simulink model "Drone_old"  (R2021a)
settings: Solver=ode45  StartTime=0.0  StopTime=20  RelTol=1e-3
values from neighbouring files (symbols this model uses):
  B = 0.001    [Params.m]
  g = 9.81    [Params.m]
  I = [I_xx 0 0; 0 I_yy 0; 0 0 I_zz]    [Params.m]
  I_xx = 3*10^(-6)    (= 3e-06)    [Params.m]
  I_yy = 3*10^(-6)    (= 3e-06)    [Params.m]
  I_zz = 1*10^(-5)    (= 1e-05)    [Params.m]
  k = 0.01    [Params.m]
  kd = 0.01    [Params.m]
  kp_h = 218.061061208643    (= 218.061061209)    [Params.m]
  kp_r = 0.0160130109024398    (= 0.0160130109024)    [Params.m]    (also in pidsolver.m = kp)
  l = 0.225    [Params.m]
  m = 0.5    [Params.m]
  tau_d_h = 44.6853606001277    (= 44.6853606001)    [Params.m]
  tau_d_r = 0.00653126952336714    (= 0.00653126952337)    [Params.m]    (also in pidsolver.m = tau_i)
  tau_i_h = 110.138309959241    (= 110.138309959)    [Params.m]
  tau_i_r = 0.00736804577025044    (= 0.00736804577025)    [Params.m]    (also in pidsolver.m = tau_i)
  w_hover = 7.830229882    [Params.m]
libraries: pid_lib x1, vrlib x1
settings Model: Creator=Marcus  LastModifiedBy=Marcus

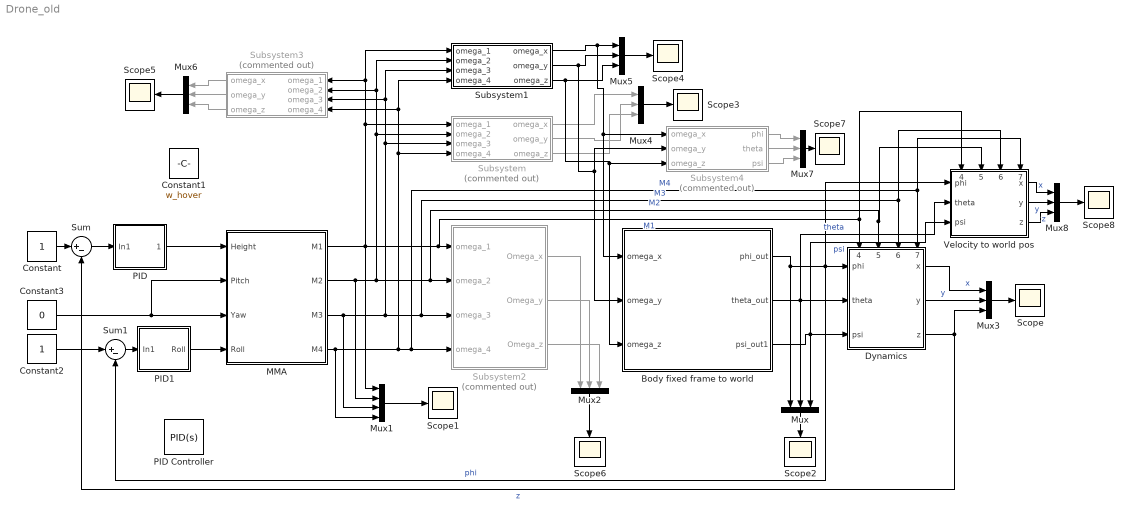
== system Drone_old ==
  Body fixed frame to world : Subsystem
  Constant : Constant  SampleTime=0.02
  Constant1 : Constant  Value=w_hover
  Constant2 : Constant  SampleTime=0.02
  Constant3 : Constant  Value=0  SampleTime=0.02
  Dynamics : Subsystem
      settings: PortSchema="{\"entries\":[{\"content\":{\"sides\":[{\"content\":{\"connectorIds\":[\"In1\",\"In2\",\"In3\"]},\"type\":\"ConnectorPlacement.EquallySpacedRectSide\",\"uuid\":\"56efaa7c-52a2-4b92-9bf3-e77850251265\"},{\"content\":{\"connectorIds\":[\"Out1\",\"Out2\",\"Out3\"],\"side\":\"RIGHT\"},\"type\":\"ConnectorPlacement.EquallySpacedRectSide\",\"uuid\":\"60524467-1949-4cc2-aa81-2e6d1e137057\"},{\"content\":{\"connectorIds\":[\"In4\",\"In5\",\"In6\",\"In7\"],\"side\":\"TOP\"},\"type\":\"ConnectorPlacement.EquallySpacedRectSide\",\"uuid\":\"33c04961-8bd6-41a2-b762-88d931b05d2b\"},{\"content\":{\"connectorIds\":[],\"side\":\"BOTTOM\"},\"type\":\"ConnectorPlacement.EquallySpacedRectSide\",\"uuid\":\"e0b8ebeb-9596-486e-9ed8-6640ac8c0b72\"}]},\"type\":\"ConnectorPlacement.EquallySpacedConnector\",\"uuid\":\"36d70e4f-9f0c-4c3e-93dc-a7f10cedf419\"}],\"packageUris\":[\"http://schema.mathworks.com/mf0/Connector/R2020b\"],\"version\":\"1.0\"}"
  MMA : Subsystem
  Mux{,2..8} (8 alike) : Mux  Inputs=3
  Mux1 : Mux
  PID : Subsystem
  PID Controller : pid_lib/PID Controller  Controller=PID  Form=Parallel  TimeDomain=Continuous-time  UseExternalTs=off  SampleTime=-1  IntegratorMethod=Forward Euler  FilterMethod=Forward Euler  ControllerParametersSource=internal  P=0.0160130109024398  I=0.00736804577025044  D=0.00653126952336714  UseFilter=on  N=1142.8279760416  TunerSelectOption=Transfer Function Based (PID Tuner App)  InitialConditionSource=internal  InitialConditionForIntegrator=0  InitialConditionForFilter=0  DifferentiatorICPrevScaledInput=0  ExternalReset=none  TrackingMode=off  Kt=1  LimitOutput=off  SatLimitsSource=internal  UpperSaturationLimit=inf  LowerSaturationLimit=-inf  LinearizeAsGain=on  AntiWindupMode=none  Kb=1  POutMin=[]  POutMax=[]  IOutMin=[]  IOutMax=[]  DOutMin=[]  DOutMax=[]  NOutMin=[]  NOutMax=[]  SumOutMin=[]  SumOutMax=[]  SaturationOutMin=[]  SaturationOutMax=[]  PParamMin=[]  PParamMax=[]  IParamMin=[]  IParamMax=[]  DParamMin=[]  DParamMax=[]  NParamMin=[]  NParamMax=[]  KbParamMin=[]  KbParamMax=[]  KtParamMin=[]  KtParamMax=[]  KbOutMin=[]  KbOutMax=[]  KtOutMin=[]  KtOutMax=[]  IntegratorOutMin=[]  IntegratorOutMax=[]  FilterOutMin=[]  FilterOutMax=[]  SumI1OutMin=[]  SumI1OutMax=[]  SumI2OutMin=[]  SumI2OutMax=[]  SumI3OutMin=[]  SumI3OutMax=[]  SumI4OutMin=[]  SumI4OutMax=[]  SumDOutMin=[]  SumDOutMax=[]  DifferentiatorOutMin=[]  DifferentiatorOutMax=[]  FilterDiffOutCoefMin=[]  FilterDiffOutCoefMax=[]  ReciprocalOutMin=[]  ReciprocalOutMax=[]  SumDenOutMin=[]  SumDenOutMax=[]  SumNumOutMin=[]  SumNumOutMax=[]  DivideOutMin=[]  DivideOutMax=[]  UdiffTsProdOutMin=[]  UdiffTsProdOutMax=[]  NTsProdOutMin=[]  NTsProdOutMax=[]  UintegralTsProdOutMin=[]  UintegralTsProdOutMax=[]  UngainTsProdOutMin=[]  UngainTsProdOutMax=[]  IntegratorContinuousStateAttributes=''  IntegratorStateMustResolveToSignalObject=off  IntegratorRTWStateStorageClass=Auto  FilterContinuousStateAttributes=''  FilterStateMustResolveToSignalObject=off  FilterRTWStateStorageClass=Auto  ParallelPVariant=InternalParameters  IdealPVariant=Disabled  IVariant=InternalParameters  DVariant=InternalParameters  IntegratorVariant=Continuous  SatVariant=Disabled  AWVariant=Passthrough  PCopyVariant=Disabled  TRVariant=Disabled  FdbkBlocksVariant=Forward  IdealPFdbkVariant=Disabled  SatFdbkVariant=Disabled  DerivativeFilterVariant=ContFilter  NVariant=InternalParameters  NCopyVariant=Disabled  FilterICVariant=InternalICsFilter  IntegratorICVariant=InternalICs  ExternalResetVariant=Disabled  TRSumVariant=Passthrough  SumFdbkVariant=Disabled  SumVariant=Sum_PID  TsampFilterVariant=InternalTs  TsampNgainVariant=Passthrough  TsampIntegralVariant=Passthrough  ExternalSaturationOutDataTypeStr=Inherit: Same as second input
  PID1 : Subsystem
  Scope{,1..8} (9 alike) : Scope
  Subsystem : Subsystem  Commented=on
  Subsystem1 : Subsystem
  Subsystem2 : Subsystem  Commented=on
  Subsystem3 : Subsystem  Commented=on
  Subsystem4 : Subsystem  Commented=on
  Sum : Sum  Inputs=|+-
  Sum1 : Sum  Inputs=|+-
  Velocity to world pos : Subsystem
      settings: PortSchema="{\"entries\":[{\"content\":{\"sides\":[{\"content\":{\"connectorIds\":[\"In1\",\"In2\",\"In3\"]},\"type\":\"ConnectorPlacement.EquallySpacedRectSide\",\"uuid\":\"56efaa7c-52a2-4b92-9bf3-e77850251265\"},{\"content\":{\"connectorIds\":[\"Out1\",\"Out2\",\"Out3\"],\"side\":\"RIGHT\"},\"type\":\"ConnectorPlacement.EquallySpacedRectSide\",\"uuid\":\"60524467-1949-4cc2-aa81-2e6d1e137057\"},{\"content\":{\"connectorIds\":[\"In4\",\"In5\",\"In6\",\"In7\"],\"side\":\"TOP\"},\"type\":\"ConnectorPlacement.EquallySpacedRectSide\",\"uuid\":\"33c04961-8bd6-41a2-b762-88d931b05d2b\"},{\"content\":{\"connectorIds\":[],\"side\":\"BOTTOM\"},\"type\":\"ConnectorPlacement.EquallySpacedRectSide\",\"uuid\":\"e0b8ebeb-9596-486e-9ed8-6640ac8c0b72\"}]},\"type\":\"ConnectorPlacement.EquallySpacedConnector\",\"uuid\":\"36d70e4f-9f0c-4c3e-93dc-a7f10cedf419\"}],\"packageUris\":[\"http://schema.mathworks.com/mf0/Connector/R2020b\"],\"version\":\"1.0\"}"
  wires:
  Body fixed frame to world/2(theta_out) -> Velocity to world pos/2(theta), Dynamics/2(theta), Mux/2  "theta"
  Subsystem2/3(Omega_z) -> Mux2/3
  Body fixed frame to world/1(phi_out) -> Mux/1, Velocity to world pos/1(phi), Sum1/2, Dynamics/1(phi)  "phi"
  Subsystem2/1(Omega_x) -> Mux2/1
  Body fixed frame to world/3(psi_out1) -> Velocity to world pos/3(psi), Dynamics/3(psi), Mux/3  "psi"
  Subsystem2/2(Omega_y) -> Mux2/2
  MMA/1(M1) -> Subsystem3/1(omega_1), Subsystem1/1(omega_1), Subsystem/1(omega_1), Dynamics/4(Input), Velocity to world pos/4(Input), Subsystem2/1(omega_1), Mux1/1  "M1"
  MMA/2(M2) -> Mux1/2, Subsystem3/2(omega_2), Subsystem1/2(omega_2), Subsystem/2(omega_2), Velocity to world pos/5(Input1), Dynamics/5(Input1), Subsystem2/2(omega_2)  "M2"
  MMA/3(M3) -> Mux1/3, Subsystem3/3(omega_3), Subsystem1/3(omega_3), Subsystem/3(omega_3), Subsystem2/3(omega_3), Dynamics/6(Input2), Velocity to world pos/6(Input2)  "M3"
  MMA/4(M4) -> Mux1/4, Subsystem3/4(omega_4), Subsystem1/4(omega_4), Subsystem/4(omega_4), Dynamics/7(Input3), Velocity to world pos/7(Input3), Subsystem2/4(omega_4)  "M4"
  Mux/1 -> Scope2/1
  Mux1/1 -> Scope1/1
  Constant/1 -> Sum/1
  Dynamics/2(y) -> Mux3/2  "y"
  Dynamics/1(x) -> Mux3/1  "x"
  Mux3/1 -> Scope/1
  Mux2/1 -> Scope6/1
  Subsystem/1(omega_x) -> Mux4/1
  Subsystem/2(omega_y) -> Mux4/2
  Subsystem/3(omega_z) -> Mux4/3
  Mux4/1 -> Scope3/1
  Mux5/1 -> Scope4/1
  Subsystem1/1(omega_x) -> Body fixed frame to world/1(omega_x), Subsystem4/1(omega_x), Mux5/1
  Subsystem1/2(omega_y) -> Body fixed frame to world/2(omega_y), Subsystem4/2(omega_y), Mux5/2
  Subsystem1/3(omega_z) -> Body fixed frame to world/3(omega_z), Subsystem4/3(omega_z), Mux5/3
  Mux6/1 -> Scope5/1
  Subsystem3/1(omega_x) -> Mux6/1
  Subsystem3/2(omega_y) -> Mux6/2
  Subsystem3/3(omega_z) -> Mux6/3
  Subsystem4/1(phi) -> Mux7/1
  Subsystem4/2(theta) -> Mux7/2
  Subsystem4/3(psi) -> Mux7/3
  Mux7/1 -> Scope7/1
  Dynamics/3(z) -> Sum/2, Mux3/3  "z"
  Constant2/1 -> Sum1/1
  Sum1/1 -> PID1/1(In1)
  PID1/1(Roll) -> MMA/4(Roll)
  Sum/1 -> PID/1(In1)
  PID/1(Height) -> MMA/1(Height)
  Mux8/1 -> Scope8/1
  Velocity to world pos/1(x) -> Mux8/1  "x"
  Velocity to world pos/2(y) -> Mux8/2  "y"
  Velocity to world pos/3(z) -> Mux8/3  "z"
  Constant3/1 -> MMA/2(Pitch), MMA/3(Yaw)

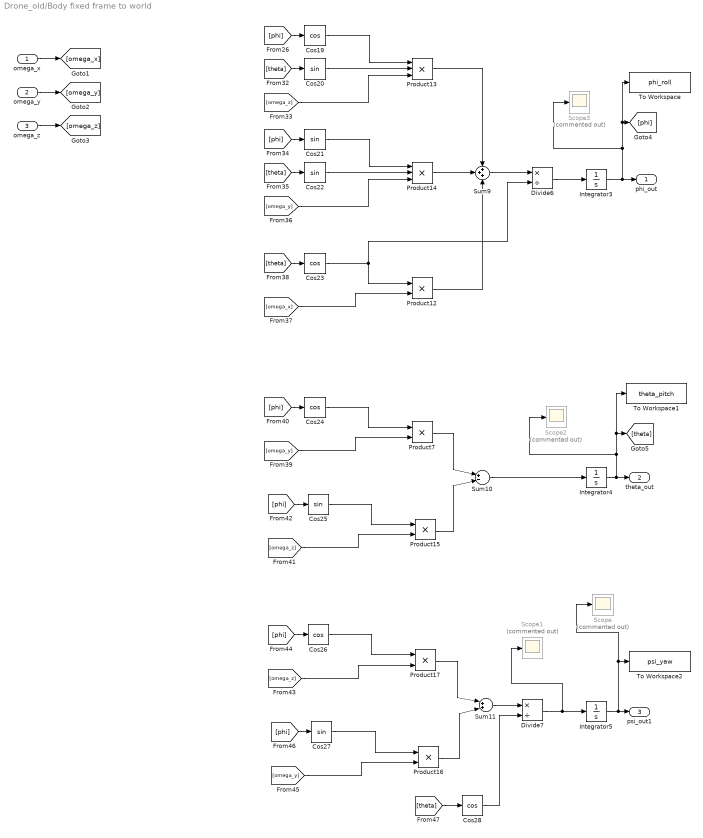
== system Drone_old/Body fixed frame to world ==
  omega_x : Inport
  omega_y : Inport  Port=2
  omega_z : Inport  Port=3
  Cos{19,23..24,26,28} (5 alike) : Trigonometry  Operator=cos
  Cos{20..22,25,27} (5 alike) : Trigonometry
  Divide6 : Product  Inputs=*/
  Divide7 : Product  Inputs=*/
  Integrator3 : Integrator
  Integrator4 : Integrator
  Integrator5 : Integrator
  Product{7,12,15..17} (5 alike) : Product
  Product13 : Product  Inputs=3
  Product14 : Product  Inputs=3
  Scope{,1..3} (4 alike) : Scope  Commented=on
  Sum10 : Sum  Inputs=|+-|
  Sum11 : Sum  Inputs=|++|
  Sum9 : Sum  Inputs=+++
  To Workspace : ToWorkspace  VariableName=phi_roll  SaveFormat=Timeseries  SampleTime=-1
  To Workspace1 : ToWorkspace  VariableName=theta_pitch  SaveFormat=Timeseries  SampleTime=-1
  To Workspace2 : ToWorkspace  VariableName=psi_yaw  SaveFormat=Timeseries  SampleTime=-1
  phi_out : Outport
  theta_out : Outport  Port=2
  psi_out1 : Outport  Port=3
  wires:
  omega_x/1 -> [omega_x]
  omega_y/1 -> [omega_y]
  omega_z/1 -> [omega_z]
  Cos19/1 -> Product13/1
  [phi] -> Cos19/1
  Cos20/1 -> Product13/2
  [theta] -> Cos20/1
  [omega_z] -> Product13/3
  Cos22/1 -> Product14/2
  [theta] -> Cos22/1
  [phi] -> Cos21/1
  Cos21/1 -> Product14/1
  [omega_y] -> Product14/3
  [omega_x] -> Product12/2
  [theta] -> Cos23/1
  Cos23/1 -> Product12/1, Divide6/2
  Product14/1 -> Sum9/2
  Product13/1 -> Sum9/1
  Product12/1 -> Sum9/3
  Sum9/1 -> Divide6/1
  Divide6/1 -> Integrator3/1
  Integrator3/1 -> Scope3/1, To Workspace/1, [phi], phi_out/1
  [omega_y] -> Product7/2
  Cos24/1 -> Product7/1
  [phi] -> Cos24/1
  [phi] -> Cos25/1
  Cos25/1 -> Product15/1
  [omega_z] -> Product15/2
  Product15/1 -> Sum10/2
  Product7/1 -> Sum10/1
  Sum10/1 -> Integrator4/1
  Integrator4/1 -> Scope2/1, To Workspace1/1, [theta], theta_out/1
  Product17/1 -> Sum11/1
  [phi] -> Cos26/1
  [omega_z] -> Product17/2
  Cos27/1 -> Product16/1
  [phi] -> Cos27/1
  Integrator5/1 -> Scope/1, To Workspace2/1, psi_out1/1
  [omega_y] -> Product16/2
  Cos26/1 -> Product17/1
  Product16/1 -> Sum11/2
  Sum11/1 -> Divide7/1
  Cos28/1 -> Divide7/2
  [theta] -> Cos28/1
  Divide7/1 -> Scope1/1, Integrator5/1

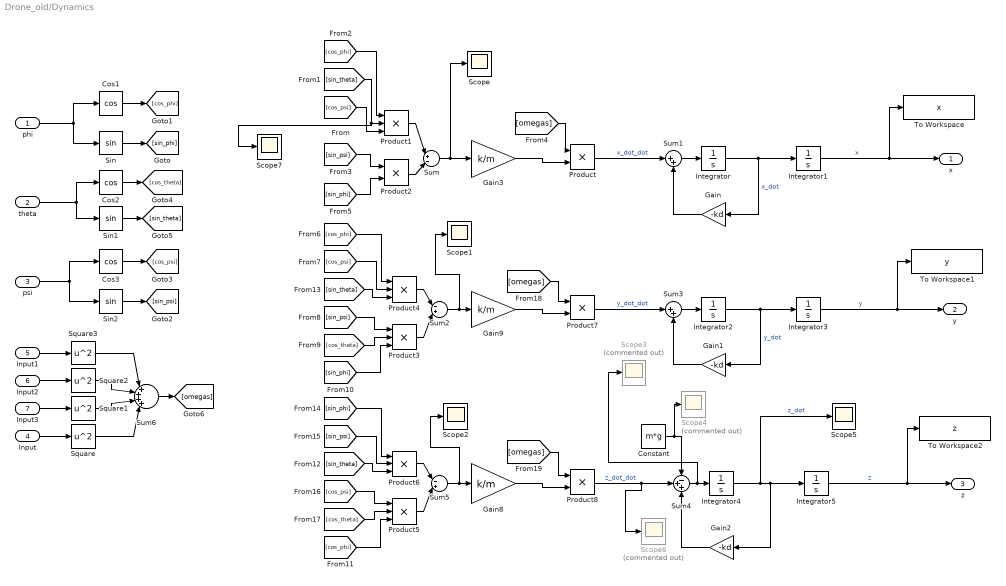
== system Drone_old/Dynamics ==
  phi : Inport
  theta : Inport  Port=2
  psi : Inport  Port=3
  Input : Inport  Port=4
  Input1 : Inport  Port=5
  Input2 : Inport  Port=6
  Input3 : Inport  Port=7
  Constant : Constant  Value=m*g
  Cos1 : Trigonometry  Operator=cos
  Cos2 : Trigonometry  Operator=cos
  Cos3 : Trigonometry  Operator=cos
  Gain : Gain  Gain=-kd
  Gain1 : Gain  Gain=-kd
  Gain2 : Gain  Gain=-kd
  Gain3 : Gain  Gain=k/m
  Gain8 : Gain  Gain=k/m
  Gain9 : Gain  Gain=k/m
  Integrator : Integrator  ZeroCross=off
  Integrator{1..5} (5 alike) : Integrator
  Product{,2,7..8} (4 alike) : Product
  Product{1,3..6} (5 alike) : Product  Inputs=3
  Scope{,1..2,5,7} (5 alike) : Scope
  Scope3 : Scope  Commented=on
  Scope4 : Scope  Commented=on
  Scope6 : Scope  Commented=on
  Sin : Trigonometry
  Sin1 : Trigonometry
  Sin2 : Trigonometry
  Square{,1..3} (4 alike) : Math  Operator=square  SaturateOnIntegerOverflow=on
  Sum : Sum  Inputs=|+-|
  Sum1 : Sum  Inputs=|++
  Sum2 : Sum  Inputs=|-+|
  Sum3 : Sum  Inputs=|++
  Sum4 : Sum  Inputs=-++
  Sum5 : Sum  Inputs=|-+|
  Sum6 : Sum  Inputs=|++++|
  To Workspace : ToWorkspace  VariableName=x  SaveFormat=Timeseries  SampleTime=-1
  To Workspace1 : ToWorkspace  VariableName=y  SaveFormat=Timeseries  SampleTime=-1
  To Workspace2 : ToWorkspace  VariableName=z  SaveFormat=Timeseries  SampleTime=-1
  x : Outport
  y : Outport  Port=2
  z : Outport  Port=3
  wires:
  Gain/1 -> Sum1/2
  Integrator5/1 -> z/1, To Workspace2/1  "z"
  [cos_phi] -> Product4/1
  Product2/1 -> Sum/2
  [sin_psi] -> Product3/1
  Sum1/1 -> Integrator/1
  Sum/1 -> Scope/1, Gain3/1
  [sin_theta] -> Scope7/1, Product1/2
  phi/1 -> Cos1/1, Sin/1
  Gain1/1 -> Sum3/2
  Integrator3/1 -> y/1, To Workspace1/1  "y"
  [sin_psi] -> Product2/1
  Product3/1 -> Sum2/2
  Integrator2/1 -> Gain1/1, Integrator3/1  "y_dot"
  psi/1 -> Sin2/1, Cos3/1
  [cos_phi] -> Product5/3
  Cos2/1 -> [cos_theta]
  [sin_theta] -> Product6/3
  [cos_psi] -> Product1/3
  Integrator1/1 -> x/1, To Workspace/1  "x"
  Sum3/1 -> Integrator2/1
  Sum5/1 -> Scope2/1, Gain8/1
  Product/1 -> Sum1/1  "x_dot_dot"
  Integrator4/1 -> Scope5/1, Gain2/1, Integrator5/1  "z_dot"
  [sin_phi] -> Product3/3
  [cos_psi] -> Product4/2
  Product1/1 -> Sum/1
  Cos3/1 -> [cos_psi]
  [cos_psi] -> Product5/1
  [sin_psi] -> Product6/2
  [cos_phi] -> Product1/1
  Product6/1 -> Sum5/1
  Product5/1 -> Sum5/2
  Gain3/1 -> Product/2
  Integrator/1 -> Gain/1, Integrator1/1  "x_dot"
  Sin1/1 -> [sin_theta]
  Sum2/1 -> Scope1/1, Gain9/1
  [sin_theta] -> Product4/3
  [sin_phi] -> Product6/1
  [cos_theta] -> Product5/2
  Sin2/1 -> [sin_psi]
  Cos1/1 -> [cos_phi]
  theta/1 -> Cos2/1, Sin1/1
  [cos_theta] -> Product3/2
  Sum4/1 -> Scope3/1, Integrator4/1
  Gain2/1 -> Sum4/3
  Product4/1 -> Sum2/1
  Constant/1 -> Scope4/1, Sum4/1
  Sin/1 -> [sin_phi]
  [sin_phi] -> Product2/2
  Input/1 -> Square/1
  Input3/1 -> Square1/1
  Input2/1 -> Square2/1
  Input1/1 -> Square3/1
  Square/1 -> Sum6/4
  Square1/1 -> Sum6/3
  Square2/1 -> Sum6/2
  Square3/1 -> Sum6/1
  [omegas] -> Product/1
  [omegas] -> Product7/1
  Product7/1 -> Sum3/1  "y_dot_dot"
  Gain9/1 -> Product7/2
  [omegas] -> Product8/1
  Gain8/1 -> Product8/2
  Product8/1 -> Scope6/1, Sum4/2  "z_dot_dot"
  Sum6/1 -> [omegas]

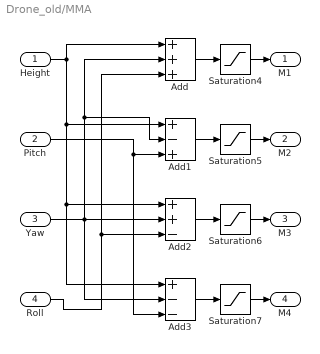
== system Drone_old/MMA ==
  Height : Inport
  Pitch : Inport  Port=2
  Yaw : Inport  Port=3
  Roll : Inport  Port=4
  Add : Sum  Inputs=+++
  Add1 : Sum  Inputs=+-+
  Add2 : Sum  Inputs=++-
  Add3 : Sum  Inputs=+--
  Saturation{4..7} (4 alike) : Saturate  UpperLimit=20000  LowerLimit=0  ZeroCross=off
  M1 : Outport
  M2 : Outport  Port=2
  M3 : Outport  Port=3
  M4 : Outport  Port=4
  wires:
  Height/1 -> Add3/1, Add2/1, Add1/1, Add/1
  Pitch/1 -> Add3/3, Add1/3
  Yaw/1 -> Add3/2, Add2/2, Add/2, Add1/2
  Roll/1 -> Add2/3, Add/3
  Add2/1 -> Saturation6/1
  Add3/1 -> Saturation7/1
  Add1/1 -> Saturation5/1
  Add/1 -> Saturation4/1
  Saturation4/1 -> M1/1
  Saturation5/1 -> M2/1
  Saturation6/1 -> M3/1
  Saturation7/1 -> M4/1

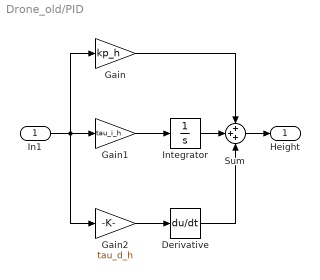
== system Drone_old/PID ==
  In1 : Inport
  Derivative : Derivative
  Gain : Gain  Gain=kp_h
  Gain1 : Gain  Gain=tau_i_h
  Gain2 : Gain  Gain=tau_d_h
  Integrator : Integrator
  Sum : Sum  Inputs=+++
  Height : Outport
  wires:
  In1/1 -> Gain2/1, Gain1/1, Gain/1
  Gain1/1 -> Integrator/1
  Integrator/1 -> Sum/2
  Gain2/1 -> Derivative/1
  Sum/1 -> Height/1
  Gain/1 -> Sum/1
  Derivative/1 -> Sum/3

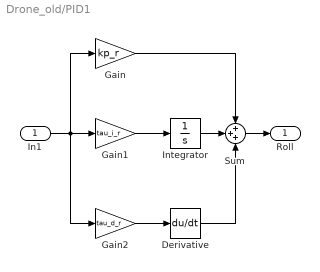
== system Drone_old/PID1 ==
  In1 : Inport
  Derivative : Derivative
  Gain : Gain  Gain=kp_r
  Gain1 : Gain  Gain=tau_i_r
  Gain2 : Gain  Gain=tau_d_r
  Integrator : Integrator
  Sum : Sum  Inputs=+++
  Roll : Outport
  wires:
  In1/1 -> Gain2/1, Gain1/1, Gain/1
  Gain1/1 -> Integrator/1
  Integrator/1 -> Sum/2
  Gain2/1 -> Derivative/1
  Sum/1 -> Roll/1
  Gain/1 -> Sum/1
  Derivative/1 -> Sum/3

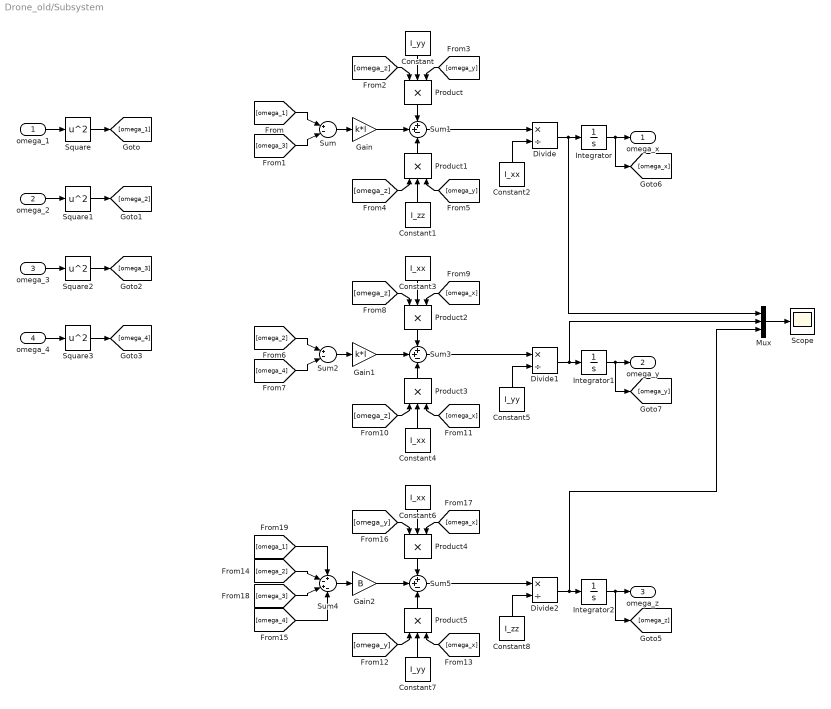
== system Drone_old/Subsystem ==
  omega_1 : Inport
  omega_2 : Inport  Port=2
  omega_3 : Inport  Port=3
  omega_4 : Inport  Port=4
  Constant : Constant  Value=I_yy
  Constant1 : Constant  Value=I_zz
  Constant{2..4,6} (4 alike) : Constant  Value=I_xx
  Constant5 : Constant  Value=I_yy
  Constant7 : Constant  Value=I_yy
  Constant8 : Constant  Value=I_zz
  Divide : Product  Inputs=*/
  Divide1 : Product  Inputs=*/
  Divide2 : Product  Inputs=*/
  Gain : Gain  Gain=k*l
  Gain1 : Gain  Gain=k*l
  Gain2 : Gain  Gain=B
  Integrator : Integrator
  Integrator1 : Integrator
  Integrator2 : Integrator
  Mux : Mux  Inputs=3
  Product{,1..5} (6 alike) : Product  Inputs=3
  Scope : Scope
  Square{,1..3} (4 alike) : Math  Operator=square  SaturateOnIntegerOverflow=on
  Sum : Sum  Inputs=|+-|
  Sum1 : Sum  Inputs=++-
  Sum2 : Sum  Inputs=|+-|
  Sum3 : Sum  Inputs=++-
  Sum4 : Sum  Inputs=+-+-
  Sum5 : Sum  Inputs=++-
  omega_x : Outport
  omega_y : Outport  Port=2
  omega_z : Outport  Port=3
  wires:
  omega_1/1 -> Square/1
  omega_2/1 -> Square1/1
  omega_3/1 -> Square2/1
  omega_4/1 -> Square3/1
  Square/1 -> [omega_1]
  Square1/1 -> [omega_2]
  Square2/1 -> [omega_3]
  Square3/1 -> [omega_4]
  [omega_1] -> Sum/1
  [omega_3] -> Sum/2
  Sum/1 -> Gain/1
  Gain/1 -> Sum1/2
  Product/1 -> Sum1/1
  [omega_z] -> Product/1
  [omega_y] -> Product/3
  Constant/1 -> Product/2
  [omega_z] -> Product1/1
  [omega_y] -> Product1/3
  Constant1/1 -> Product1/2
  Product1/1 -> Sum1/3
  Sum1/1 -> Divide/1
  Constant2/1 -> Divide/2
  Divide/1 -> Mux/1, Integrator/1
  Integrator/1 -> [omega_x], omega_x/1
  Sum3/1 -> Divide1/1
  [omega_z] -> Product2/1
  [omega_4] -> Sum2/2
  Integrator1/1 -> [omega_y], omega_y/1
  Divide1/1 -> Mux/2, Integrator1/1
  Product3/1 -> Sum3/3
  Constant5/1 -> Divide1/2
  Product2/1 -> Sum3/1
  [omega_x] -> Product2/3
  Constant3/1 -> Product2/2
  Constant4/1 -> Product3/2
  [omega_z] -> Product3/1
  Gain1/1 -> Sum3/2
  [omega_x] -> Product3/3
  [omega_2] -> Sum2/1
  Sum2/1 -> Gain1/1
  [omega_x] -> Product5/3
  [omega_2] -> Sum4/2
  Sum4/1 -> Gain2/1
  Gain2/1 -> Sum5/2
  Constant6/1 -> Product4/2
  [omega_y] -> Product5/1
  Constant7/1 -> Product5/2
  Constant8/1 -> Divide2/2
  Product4/1 -> Sum5/1
  [omega_x] -> Product4/3
  Product5/1 -> Sum5/3
  Divide2/1 -> Mux/3, Integrator2/1
  Sum5/1 -> Divide2/1
  [omega_y] -> Product4/1
  [omega_4] -> Sum4/4
  Integrator2/1 -> [omega_z], omega_z/1
  [omega_3] -> Sum4/3
  [omega_1] -> Sum4/1
  Mux/1 -> Scope/1

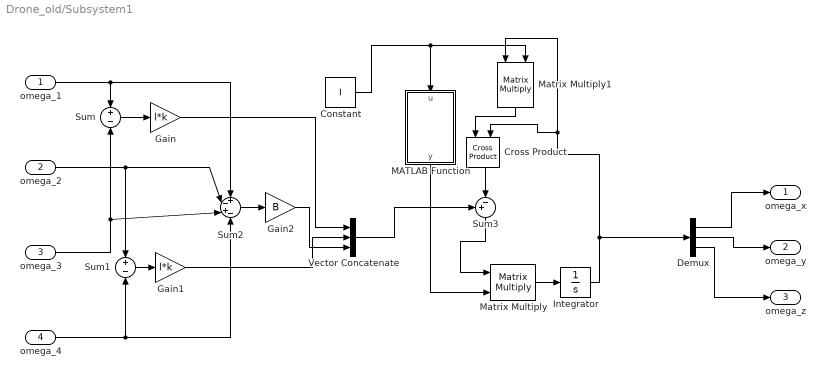
== system Drone_old/Subsystem1 ==
  omega_1 : Inport
  omega_2 : Inport  Port=2
  omega_3 : Inport  Port=3
  omega_4 : Inport  Port=4
  Constant : Constant  Value=I
  Cross Product : vrlib/Utilities/Cross Product
  Demux : Demux  Outputs=3
  Gain : Gain  Gain=l*k
  Gain1 : Gain  Gain=l*k
  Gain2 : Gain  Gain=B
  Integrator : Integrator
  MATLAB Function : MATLAB Function  TreatAsAtomicUnit=on
  Matrix Multiply : Product  Multiplication=Matrix(*)
  Matrix Multiply1 : Product  Multiplication=Matrix(*)
  Sum : Sum  Inputs=+-
  Sum1 : Sum  Inputs=+-
  Sum2 : Sum  Inputs=+-+-
  Sum3 : Sum  Inputs=+-|
  Vector Concatenate : Concatenate  NumInputs=3
  omega_x : Outport
  omega_y : Outport  Port=2
  omega_z : Outport  Port=3
  wires:
  Integrator/1 -> Matrix Multiply1/1, Cross Product/2, Demux/1
  omega_1/1 -> Sum2/1, Sum/1
  omega_3/1 -> Sum2/3, Sum/2
  Sum/1 -> Gain/1
  omega_2/1 -> Sum2/2, Sum1/1
  omega_4/1 -> Sum1/2, Sum2/4
  Sum1/1 -> Gain1/1
  Sum2/1 -> Gain2/1
  Gain1/1 -> Vector Concatenate/2
  Gain/1 -> Vector Concatenate/1
  Gain2/1 -> Vector Concatenate/3
  Demux/1 -> omega_x/1
  Demux/2 -> omega_y/1
  Demux/3 -> omega_z/1
  Constant/1 -> Matrix Multiply1/2, MATLAB Function/1(u)
  Matrix Multiply1/1 -> Cross Product/1
  Cross Product/1 -> Sum3/2
  Matrix Multiply/1 -> Integrator/1
  Sum3/1 -> Matrix Multiply/1
  MATLAB Function/1(y) -> Matrix Multiply/2
  Vector Concatenate/1 -> Sum3/1

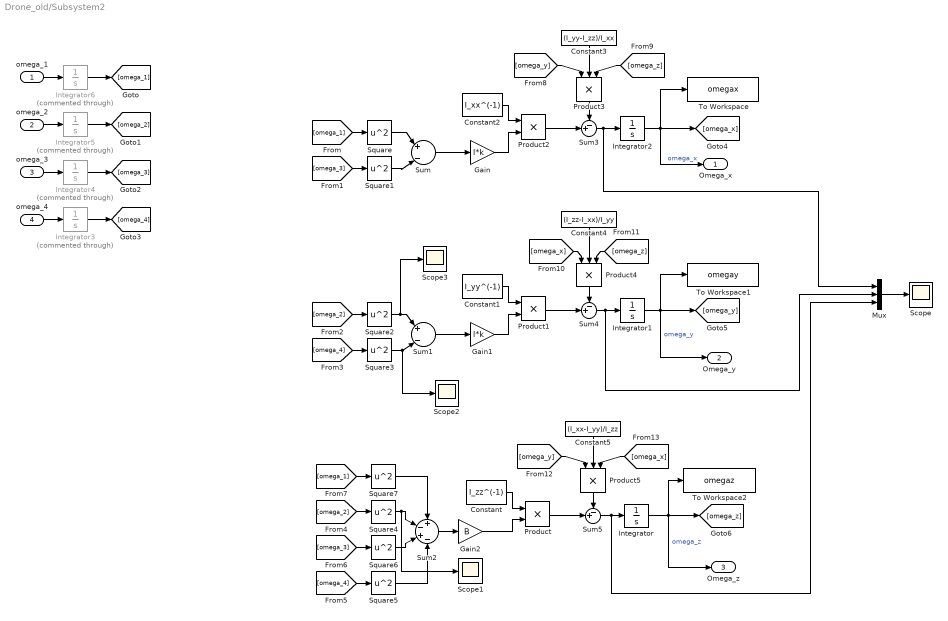
== system Drone_old/Subsystem2 ==
  omega_1 : Inport
  omega_2 : Inport  Port=2
  omega_3 : Inport  Port=3
  omega_4 : Inport  Port=4
  Constant : Constant  Value=I_zz^(-1)
  Constant1 : Constant  Value=I_yy^(-1)
  Constant2 : Constant  Value=I_xx^(-1)
  Constant3 : Constant  Value=(I_yy-I_zz)/I_xx
  Constant4 : Constant  Value=(I_zz-I_xx)/I_yy
  Constant5 : Constant  Value=(I_xx-I_yy)/I_zz
  Gain : Gain  Gain=l*k
  Gain1 : Gain  Gain=l*k
  Gain2 : Gain  Gain=B
  Integrator : Integrator
  Integrator1 : Integrator
  Integrator2 : Integrator
  Integrator{3..6} (4 alike) : Integrator  Commented=through
  Mux : Mux  Inputs=3
  Product : Product
  Product1 : Product
  Product2 : Product
  Product3 : Product  Inputs=3
  Product4 : Product  Inputs=3
  Product5 : Product  Inputs=3
  Scope{,1..3} (4 alike) : Scope
  Square{,1..7} (8 alike) : Math  Operator=square  SaturateOnIntegerOverflow=on
  Sum : Sum  Inputs=|+|-|
  Sum1 : Sum  Inputs=|+|-|
  Sum2 : Sum  Inputs=+-+-
  Sum3 : Sum  Inputs=-+|
  Sum4 : Sum  Inputs=-+|
  Sum5 : Sum  Inputs=-+|
  To Workspace : ToWorkspace  VariableName=omegax  SaveFormat=Timeseries  SampleTime=-1
  To Workspace1 : ToWorkspace  VariableName=omegay  SaveFormat=Timeseries  SampleTime=-1
  To Workspace2 : ToWorkspace  VariableName=omegaz  SaveFormat=Timeseries  SampleTime=-1
  Omega_x : Outport
  Omega_y : Outport  Port=2
  Omega_z : Outport  Port=3
  wires:
  omega_1/1 -> Integrator6/1
  omega_2/1 -> Integrator5/1
  omega_3/1 -> Integrator4/1
  omega_4/1 -> Integrator3/1
  [omega_1] -> Square/1
  Square/1 -> Sum/1
  [omega_3] -> Square1/1
  Square1/1 -> Sum/2
  Sum/1 -> Gain/1
  Square3/1 -> Scope2/1, Sum1/2
  Sum1/1 -> Gain1/1
  [omega_2] -> Square2/1
  Square2/1 -> Scope3/1, Sum1/1
  [omega_4] -> Square3/1
  Square4/1 -> Scope1/1, Sum2/2
  Sum2/1 -> Gain2/1
  Square5/1 -> Sum2/4
  [omega_4] -> Square5/1
  [omega_2] -> Square4/1
  [omega_3] -> Square6/1
  Square6/1 -> Sum2/3
  [omega_1] -> Square7/1
  Square7/1 -> Sum2/1
  Gain2/1 -> Product/2
  Constant/1 -> Product/1
  Constant1/1 -> Product1/1
  Gain1/1 -> Product1/2
  Constant2/1 -> Product2/1
  Gain/1 -> Product2/2
  Product2/1 -> Sum3/2
  Product1/1 -> Sum4/2
  Product/1 -> Sum5/2
  Sum3/1 -> Mux/1, Integrator2/1
  Sum4/1 -> Mux/2, Integrator1/1
  Integrator/1 -> To Workspace2/1, Omega_z/1, [omega_z]  "omega_z"
  Integrator1/1 -> To Workspace1/1, Omega_y/1, [omega_y]  "omega_y"
  Integrator2/1 -> To Workspace/1, Omega_x/1, [omega_x]  "omega_x"
  Product3/1 -> Sum3/1
  Constant3/1 -> Product3/2
  [omega_z] -> Product3/3
  Product4/1 -> Sum4/1
  [omega_z] -> Product4/3
  Constant4/1 -> Product4/2
  Product5/1 -> Sum5/1
  [omega_y] -> Product5/1
  [omega_x] -> Product5/3
  Constant5/1 -> Product5/2
  Sum5/1 -> Mux/3, Integrator/1
  Mux/1 -> Scope/1
  Integrator3/1 -> [omega_4]
  Integrator4/1 -> [omega_3]
  Integrator5/1 -> [omega_2]
  Integrator6/1 -> [omega_1]
  [omega_x] -> Product4/1
  [omega_y] -> Product3/1

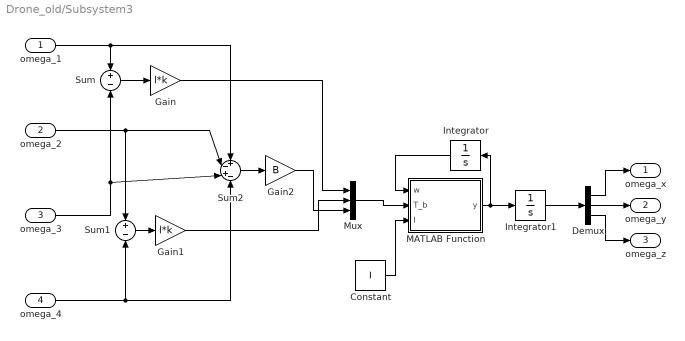
== system Drone_old/Subsystem3 ==
  omega_1 : Inport
  omega_2 : Inport  Port=2
  omega_3 : Inport  Port=3
  omega_4 : Inport  Port=4
  Constant : Constant  Value=I
  Demux : Demux  Outputs=3
  Gain : Gain  Gain=l*k
  Gain1 : Gain  Gain=l*k
  Gain2 : Gain  Gain=B
  Integrator : Integrator  InitialCondition=[0.001 0.001 0.001]
  Integrator1 : Integrator
  MATLAB Function : MATLAB Function  TreatAsAtomicUnit=on
  Mux : Mux  Inputs=3
  Sum : Sum  Inputs=+-
  Sum1 : Sum  Inputs=+-
  Sum2 : Sum  Inputs=+-+-
  omega_x : Outport
  omega_y : Outport  Port=2
  omega_z : Outport  Port=3
  wires:
  omega_1/1 -> Sum2/1, Sum/1
  omega_3/1 -> Sum2/3, Sum/2
  Sum/1 -> Gain/1
  omega_2/1 -> Sum2/2, Sum1/1
  omega_4/1 -> Sum1/2, Sum2/4
  Sum1/1 -> Gain1/1
  Sum2/1 -> Gain2/1
  Gain1/1 -> Mux/2
  Gain/1 -> Mux/1
  Gain2/1 -> Mux/3
  Mux/1 -> MATLAB Function/2(T_b)
  Constant/1 -> MATLAB Function/3(I)
  MATLAB Function/1(y) -> Integrator1/1, Integrator/1
  Integrator/1 -> MATLAB Function/1(w)
  Demux/1 -> omega_x/1
  Demux/2 -> omega_y/1
  Demux/3 -> omega_z/1
  Integrator1/1 -> Demux/1

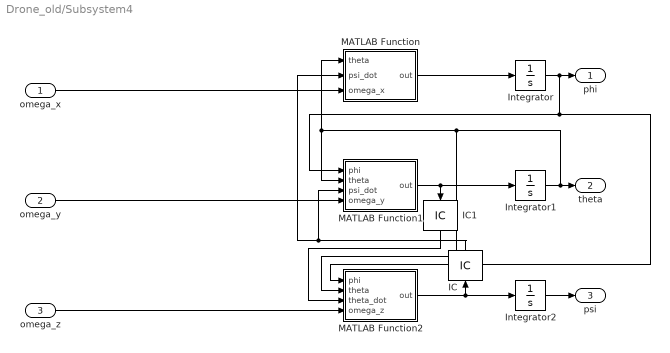
== system Drone_old/Subsystem4 ==
  omega_x : Inport
  omega_y : Inport  Port=2
  omega_z : Inport  Port=3
  IC : InitialCondition  Value=0
  IC1 : InitialCondition  Value=0
  Integrator : Integrator
  Integrator1 : Integrator
  Integrator2 : Integrator
  MATLAB Function : MATLAB Function  TreatAsAtomicUnit=on
  MATLAB Function1 : MATLAB Function  TreatAsAtomicUnit=on
  MATLAB Function2 : MATLAB Function  TreatAsAtomicUnit=on
  phi : Outport
  theta : Outport  Port=2
  psi : Outport  Port=3
  wires:
  Integrator/1 -> MATLAB Function1/1(phi), MATLAB Function2/1(phi), phi/1
  Integrator1/1 -> MATLAB Function2/2(theta), MATLAB Function1/2(theta), MATLAB Function/1(theta), theta/1
  Integrator2/1 -> psi/1
  MATLAB Function2/1(out) -> Integrator2/1, IC/1
  MATLAB Function1/1(out) -> Integrator1/1, IC1/1
  MATLAB Function/1(out) -> Integrator/1
  omega_x/1 -> MATLAB Function/3(omega_x)
  omega_y/1 -> MATLAB Function1/4(omega_y)
  omega_z/1 -> MATLAB Function2/4(omega_z)
  IC/1 -> MATLAB Function1/3(psi_dot), MATLAB Function/2(psi_dot)
  IC1/1 -> MATLAB Function2/3(theta_dot)

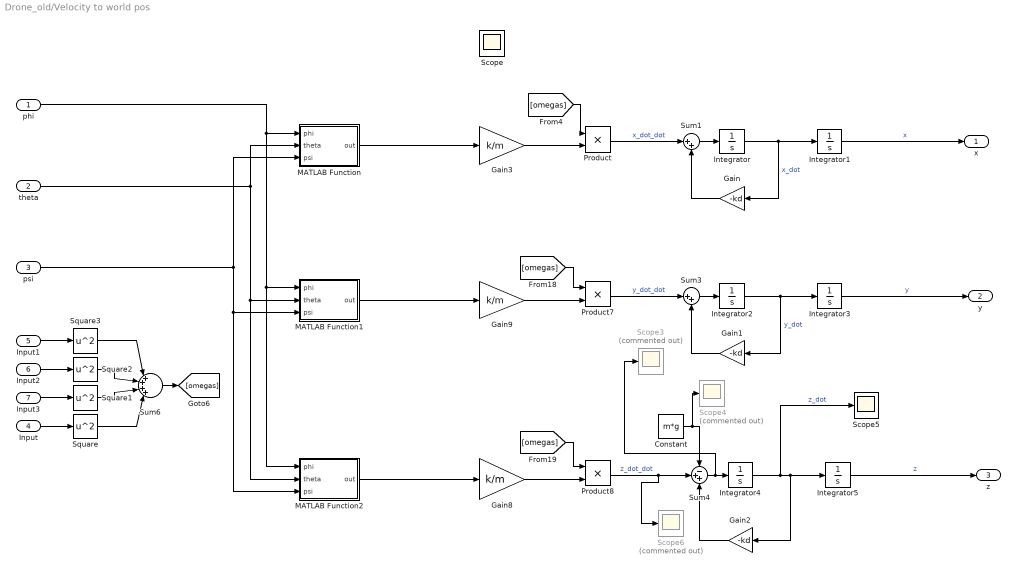
== system Drone_old/Velocity to world pos ==
  phi : Inport
  theta : Inport  Port=2
  psi : Inport  Port=3
  Input : Inport  Port=4
  Input1 : Inport  Port=5
  Input2 : Inport  Port=6
  Input3 : Inport  Port=7
  Constant : Constant  Value=m*g
  Gain : Gain  Gain=-kd
  Gain1 : Gain  Gain=-kd
  Gain2 : Gain  Gain=-kd
  Gain3 : Gain  Gain=k/m
  Gain8 : Gain  Gain=k/m
  Gain9 : Gain  Gain=k/m
  Integrator : Integrator  ZeroCross=off
  Integrator{1..5} (5 alike) : Integrator
  MATLAB Function : MATLAB Function  TreatAsAtomicUnit=on
  MATLAB Function1 : MATLAB Function  TreatAsAtomicUnit=on
  MATLAB Function2 : MATLAB Function  TreatAsAtomicUnit=on
  Product : Product
  Product7 : Product
  Product8 : Product
  Scope : Scope
  Scope3 : Scope  Commented=on
  Scope4 : Scope  Commented=on
  Scope5 : Scope
  Scope6 : Scope  Commented=on
  Square{,1..3} (4 alike) : Math  Operator=square  SaturateOnIntegerOverflow=on
  Sum1 : Sum  Inputs=|++
  Sum3 : Sum  Inputs=|++
  Sum4 : Sum  Inputs=-++
  Sum6 : Sum  Inputs=|++++|
  x : Outport
  y : Outport  Port=2
  z : Outport  Port=3
  wires:
  Gain/1 -> Sum1/2
  Integrator5/1 -> z/1  "z"
  Sum1/1 -> Integrator/1
  phi/1 -> MATLAB Function2/1(phi), MATLAB Function1/1(phi), MATLAB Function/1(phi)
  Gain1/1 -> Sum3/2
  Integrator3/1 -> y/1  "y"
  Integrator2/1 -> Gain1/1, Integrator3/1  "y_dot"
  psi/1 -> MATLAB Function/3(psi), MATLAB Function2/3(psi), MATLAB Function1/3(psi)
  Integrator1/1 -> x/1  "x"
  Sum3/1 -> Integrator2/1
  Product/1 -> Sum1/1  "x_dot_dot"
  Integrator4/1 -> Scope5/1, Gain2/1, Integrator5/1  "z_dot"
  Gain3/1 -> Product/2
  Integrator/1 -> Gain/1, Integrator1/1  "x_dot"
  theta/1 -> MATLAB Function/2(theta), MATLAB Function2/2(theta), MATLAB Function1/2(theta)
  Sum4/1 -> Scope3/1, Integrator4/1
  Gain2/1 -> Sum4/3
  Constant/1 -> Scope4/1, Sum4/1
  Input/1 -> Square/1
  Input3/1 -> Square1/1
  Input2/1 -> Square2/1
  Input1/1 -> Square3/1
  Square/1 -> Sum6/4
  Square1/1 -> Sum6/3
  Square2/1 -> Sum6/2
  Square3/1 -> Sum6/1
  [omegas] -> Product/1
  [omegas] -> Product7/1
  Product7/1 -> Sum3/1  "y_dot_dot"
  Gain9/1 -> Product7/2
  [omegas] -> Product8/1
  Gain8/1 -> Product8/2
  Product8/1 -> Scope6/1, Sum4/2  "z_dot_dot"
  Sum6/1 -> [omegas]
  MATLAB Function/1(out) -> Gain3/1
  MATLAB Function1/1(out) -> Gain9/1
  MATLAB Function2/1(out) -> Gain8/1

== matlab function Drone_old/Subsystem3/MATLAB Function ==
  data: w input; y output; T_b input; I input
function y = fcn(w, T_b, I)
    y = inv(I) * (T_b - cross(w, (I * w)));

== matlab function Drone_old/Subsystem1/MATLAB Function ==
  data: u input; y output
function y = fcn(u)
    y = inv(u);

== matlab function Drone_old/Subsystem4/MATLAB Function ==
  data: theta input; out output; psi_dot input; omega_x input
function out = fcn(theta, psi_dot, omega_x)
    out = sin(theta) * psi_dot + omega_x;

== matlab function Drone_old/Subsystem4/MATLAB Function1 ==
  data: phi input; out output; theta input; psi_dot input; omega_y input
function out = fcn(phi, theta, psi_dot, omega_y)
    out = -(sin(phi)*cos(theta)*psi_dot-omega_y)/(cos(phi));

== matlab function Drone_old/Subsystem4/MATLAB Function2 ==
  data: phi input; out output; theta input; theta_dot input; omega_z input
function out = fcn(phi, theta, theta_dot, omega_z)
    out = (omega_z + sin(phi)*theta_dot)/(cos(phi)*cos(theta));

== matlab function Drone_old/Velocity to world pos/MATLAB Function ==
  data: phi input; out output; theta input; psi input
function out = fcn(phi, theta, psi)
    out = sin(psi)*sin(phi) + cos(psi)*sin(theta)*cos(phi);

== matlab function Drone_old/Velocity to world pos/MATLAB Function1 ==
  data: phi input; out output; theta input; psi input
function out = fcn(phi, theta, psi)
    out = (-cos(psi))*sin(phi) + sin(psi)*sin(theta)*cos(phi);

== matlab function Drone_old/Velocity to world pos/MATLAB Function2 ==
  data: phi input; out output; theta input; psi input
function out = fcn(phi, theta, psi)
    out = cos(phi)*cos(theta);
